simulink model "SimPrac"  (R2018a)
settings: Solver=VariableStepAuto  StartTime=0.0  StopTime=1.0  RelTol=1e-3
undefined symbols (not defined in the file): Kwg, Lag, Lfg, Rag, Rfg, Rng, Ufg
settings Model: Creator=dirlak  LastModifiedBy=dirlak

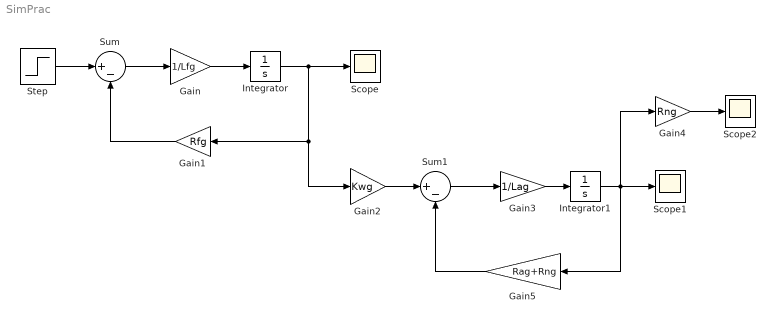
== system SimPrac ==
  Gain : Gain  Gain=1/Lfg
  Gain1 : Gain  Gain=Rfg
  Gain2 : Gain  Gain=Kwg
  Gain3 : Gain  Gain=1/Lag
  Gain4 : Gain  Gain=Rng
  Gain5 : Gain  Gain=Rag+Rng
  Integrator : Integrator
  Integrator1 : Integrator
  Scope : Scope
  Scope1 : Scope
  Scope2 : Scope
  Step : Step  Time=0  After=Ufg  SampleTime=0
  Sum : Sum  Inputs=|+-
  Sum1 : Sum  Inputs=|+-
  wires:
  Step/1 -> Sum/1
  Sum/1 -> Gain/1
  Gain/1 -> Integrator/1
  Integrator/1 -> Scope/1, Gain2/1, Gain1/1
  Gain1/1 -> Sum/2
  Gain2/1 -> Sum1/1
  Sum1/1 -> Gain3/1
  Gain3/1 -> Integrator1/1
  Integrator1/1 -> Gain4/1, Gain5/1, Scope1/1
  Gain4/1 -> Scope2/1
  Gain5/1 -> Sum1/2
